simulink model "clase05012021"  (R2020b)
settings: Solver=VariableStepAuto  StartTime=0.0  StopTime=1  RelTol=1e-3
libraries: commutil2 x1
settings Model: Creator=fernando  LastModifiedBy=fernando

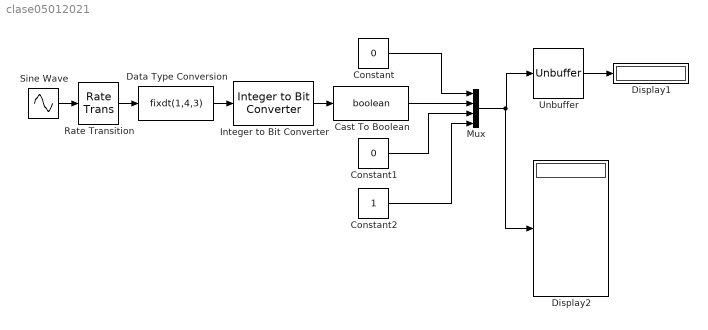
== system clase05012021 ==
  Cast To Boolean : DataTypeConversion  OutDataTypeStr=boolean
  Constant : Constant  Value=0  OutDataTypeStr=boolean
  Constant1 : Constant  Value=0  OutDataTypeStr=boolean
  Constant2 : Constant  OutDataTypeStr=boolean
  Data Type Conversion : DataTypeConversion  OutDataTypeStr=fixdt(1,4,3)
  Display1 : Display
  Display2 : Display
  Integer to Bit Converter : commutil2/Integer to Bit Converter  nbits=4  signedInputValues=Unsigned  bitOrder=MSB first  outDtype=Inherit via internal rule
  Mux : Mux
  Rate Transition : RateTransition  OutPortSampleTime=1/400
  Sine Wave : Sin  Frequency=1*pi*400  SampleTime=0
  Unbuffer : Unbuffer
  wires:
  Rate Transition/1 -> Data Type Conversion/1
  Sine Wave/1 -> Rate Transition/1
  Data Type Conversion/1 -> Integer to Bit Converter/1
  Unbuffer/1 -> Display1/1
  Mux/1 -> Display2/1, Unbuffer/1
  Integer to Bit Converter/1 -> Cast To Boolean/1
  Constant/1 -> Mux/1
  Cast To Boolean/1 -> Mux/2
  Constant1/1 -> Mux/3
  Constant2/1 -> Mux/4
